simulink model "frame_conversion"  (R2019b)
settings: Solver=FixedStepAuto  StartTime=0.0  StopTime=10.0  RelTol=1e-3
settings Model: Creator=LBRY-SVC-Patron  LastModifiedBy=logan
settings DataIOCC: ReturnWorkspaceOutputs=off
settings OptimizationCC: DefaultParameterBehavior=Inlined  UseDivisionForNetSlopeComputation=on  GainParamInheritBuiltInType=on  UseFloatMulNetSlope=on  InlineInvariantSignals=on  PassReuseOutputArgsAs=Individual arguments  ZeroExternalMemoryAtStartup=off  ZeroInternalMemoryAtStartup=off  NoFixptDivByZeroProtection=on  EfficientFloat2IntCast=on  LifeSpan=1  OptimizeBlockOrder=speed  DifferentSizesBufferReuse=on  EfficientTunableParamExpr=on
settings DebuggingCC: ParameterTunabilityLossMsg=error  ArithmeticOperatorsInVariantConditions=warning
settings HardwareCC: ProdLongLongMode=on
settings SFSimCC: SimUseLocalCustomCode=off  MATLABDynamicMemAlloc=off  CustomCodeUndefinedFunction=UseInterfaceOnly
settings RTWCC: SystemTargetFile=ert.tlc  TemplateMakefile=ert_default_tmf  GenerateReport=on  RTWUseLocalCustomCode=off  IncludeHyperlinkInReport=on  LaunchReport=on  TargetLang=C++  GenerateTraceInfo=on  GenerateTraceReport=on  GenerateTraceReportSl=on  GenerateTraceReportSf=on  GenerateTraceReportEml=on
settings CodeAppCC: ForceParamTrailComments=on  IgnoreCustomStorageClasses=off  OperatorAnnotations=on  SimulinkDataObjDesc=on  SFDataObjDesc=on  InsertBlockDesc=on
settings ERTTargetCC: TargetLangStandard=C++03 (ISO)  GenerateSampleERTMain=on  IncludeMdlTerminateFcn=off  CombineSignalStateStructs=on  MultiInstanceERTCode=on  CodeInterfacePackaging=C++ class  SupportComplex=off  SupportContinuousTime=on  InlinedParameterPlacement=NonHierarchical  RootIOFormat=Structure reference  ERTCustomFileTemplate=example_file_process.tlc  ERTFilePackagingFormat=CompactWithDataFile

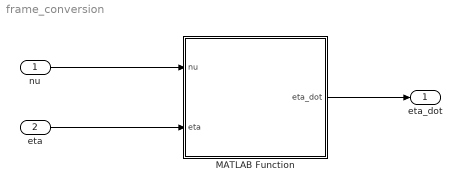
== system frame_conversion ==
  nu : Inport
  eta : Inport  Port=2
  MATLAB Function : MATLAB Function  TreatAsAtomicUnit=on
  eta_dot : Outport  PortDimensions=6  VectorParamsAs1DForOutWhenUnconnected=off
  wires:
  nu/1 -> MATLAB Function/1(nu)
  MATLAB Function/1(eta_dot) -> eta_dot/1
  eta/1 -> MATLAB Function/2(eta)

== matlab function frame_conversion/MATLAB Function ==
  data: nu input size=6; eta input size=6; eta_dot output size=6
function eta_dot = frame_converter(nu, eta)

%
% eta_dot = frame_converter(nu, eta) converts the nu vector into the 
% world frame to produce the time derivatives of the eta vector (which is 
% the position and orientation in the world frame)
%

if (length(nu) ~= 6),error('nu vector must have dimension 12 !');end
if (length(nu) ~= 6),error('eta vector must have dimension 12 !');end

phi = eta(4);      % roll angle              (rad)
theta = eta(5);    % pitch angle             (rad)
psi = eta(6);      % yaw angle               (rad)

cphi = cos(phi);
sphi = sin(phi);
cth  = cos(theta);
sth  = sin(theta);
cpsi = cos(psi);
spsi = sin(psi);

J1 = [cpsi*cth,  -spsi*cphi+cpsi*sth*sphi,   spsi*sphi+cpsi*cphi*sth; ...
      spsi*cth,   cpsi*cphi+sphi*sth*spsi,  -cpsi*sphi+sth*spsi*cphi; ...
     -sth,        cth*sphi,                  cth*cphi ];

if cth==0, error('J2 is singular for theta = +-90 degrees'); end
 
J2 = [1,  sphi*sth/cth,  cphi*sth/cth; ...
      0,  cphi,          -sphi; ...
      0,  sphi/cth,      cphi/cth ];
  
J = [ J1,  zeros(3,3); ...
      zeros(3,3), J2 ];
  
eta_dot = J*nu;
end
